simulink model "model_with_out_phases"  (R2018b)
settings: Solver=daessc  StartTime=0.0  StopTime=1  RelTol=1e-3
StopFcn:
  | % fault_type = 1005;
  | % location = 50;
  | % current = c(:,2:4);
  | % current(:,4) = fault_type;
  | % current(:,5) = location;
  | % voltage = v(:,2:4);
  | % logg = [voltage,current];
  | % data = xlsread('sdata1');
  | % data = [data;logg];
  | % xlswrite('sdata1',data);
libraries: powerlib x7, powerlib_meascontrol x2
settings Model: Creator=Edagotti Pavankumar  LastModifiedBy=Edagotti Pavankumar
settings SolverCC: ZeroCrossAlgorithm=Adaptive
settings DebuggingCC: IgnoredZcDiagnostic=none

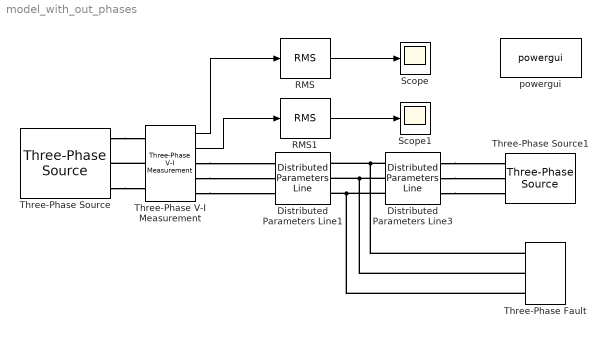
== system model_with_out_phases ==
  Distributed Parameters Line1 : powerlib/Elements/Distributed Parameters Line  Phases=3  Frequency=50  Resistance=[0.0238 0.3885]  Inductance=[0.0009509508 0.0032508989]  Capacitance=[12.74e-9 7.751e-9]  Length=50  x1=[5.84979752376728e-10 272937.603824644 272937.603824645;314.159265358979 314.159265358979 314.159265358979;1.5916152008636 0.434043679615579 -1.13675264717932]  x2=[6.54876606015739e-10 274167.064757833 274167.064757835;314.159265358979 314.159265358979 314.159265358979;1.48083589447483 0.433676655897658 -1.13711967089724]  x3=[3.33089663188176e-12 1001.56472405766 1001.56472405766;314.159265358979 314.159265358979 314.159265358979;0.373520113239949 0.324556739532956 -1.24623958726195]  x4=[1.36362276955881e-12 1001.88717060073 1001.88717060074;314.159265358979 314.159265358979 314.159265358979;2.72800603785052 0.488402443149095 -1.0823938836458]  x5=0.000250986639952707  V1=[5.85e-10 2.729e+05 2.729e+05;314.2 314.2 314.2;1.592 0.434 -1.137]  V2=[6.549e-10 2.742e+05 2.742e+05;314.2 314.2 314.2;1.481 0.4337 -1.137]  I1=[3.331e-12 1002 1002;314.2 314.2 314.2;0.3735 0.3246 -1.246]  I2=[1.364e-12 1002 1002;314.2 314.2 314.2;2.728 0.4884 -1.082]  nHarmo=1  Measurements=None
      settings: SourceProductName=Simscape Power Systems
  Distributed Parameters Line3 : powerlib/Elements/Distributed Parameters Line  Phases=3  Frequency=50  Resistance=[0.0238 0.3885]  Inductance=[0.0009509508 0.0032508989]  Capacitance=[12.74e-9 7.751e-9]  Length=150  x1=[6.54836185276508e-10 274167.064757833 274167.064757835;314.159265358979 314.159265358979 314.159265358979;1.33424699152751 0.324327959298449 -1.24646836749645]  x2=[4.51637157030593e-10 272937.917712324 272937.917712326;314.159265358979 314.159265358979 314.159265358979;1.38259637817942 0.324708516630807 -1.24608781016409]  x3=[1.33691802850131e-12 995.345525673913 995.345525673921;314.159265358979 314.159265358979 314.159265358979;2.24934769208087 0.269481792955064 -1.30131453383983]  x4=[1.38546021515408e-12 995.079620101291 995.079620101296;314.159265358979 314.159265358979 314.159265358979;0.604347333375782 0.214986476792087 -1.35580985000282]  x5=0.000752959919858122  V1=[6.548e-10 2.742e+05 2.742e+05;314.2 314.2 314.2;1.334 0.3243 -1.246]  V2=[4.516e-10 2.729e+05 2.729e+05;314.2 314.2 314.2;1.383 0.3247 -1.246]  I1=[1.337e-12 995.3 995.3;314.2 314.2 314.2;2.249 0.2695 -1.301]  I2=[1.385e-12 995.1 995.1;314.2 314.2 314.2;0.6043 0.215 -1.356]  nHarmo=1  Measurements=None
      settings: SourceProductName=Simscape Power Systems
  RMS : powerlib_meascontrol/Measurements/RMS  TrueRMS=on  Freq=50  RMSInit=0  Ts=0
  RMS1 : powerlib_meascontrol/Measurements/RMS  TrueRMS=on  Freq=50  RMSInit=0  Ts=0
  Scope : Scope
  Scope1 : Scope
  Three-Phase V-I Measurement : powerlib/Measurements/Three-Phase V-I Measurement  VoltageMeasurement=phase-to-ground  SetLabelV=off  LabelV=Vabc  Vpu=on  VpuLL=off  CurrentMeasurement=yes  SetLabelI=off  LabelI=Iabc  Ipu=on  Pbase=100e6  Vbase=220e3  OutputType=Complex  PhasorSimulation=off  PSBequivalent=0
  Three-Phase Fault : powerlib/Elements/Three-Phase Fault  InitialStates=0  FaultA=off  FaultB=on  FaultC=on  GroundFault=off  SwitchTimes=0.5  External=off  SwitchStatus=NaN  FaultResistance=20  GroundResistance=0.001  SnubberResistance=1e6  SnubberCapacitance=inf  Measurements=None
  Three-Phase Source : powerlib/Electrical Sources/Three-Phase Source  InternalConnection=Yg  VoltagePhases=off  Voltage=220e3  PhaseAngle=0  Voltage_phases=[25e3 25e3 25e3]/sqrt(3)  PhaseAngles_phases=[0 -120 +120]  Frequency=50  NonIdealSource=on  SpecifyImpedance=on  Resistance=0.8929  Inductance=16.58e-3  ShortCircuitLevel=100e6  BaseVoltage=220e3  XRratio=7  BusType=swing  Pref=10e3  Qref=0  Prefabc=[10e3, 10e3, 10e3]  Qrefabc=[0, 0, 0]  Qmin=-inf  Qmax=inf
  Three-Phase Source1 : powerlib/Electrical Sources/Three-Phase Source  InternalConnection=Yg  VoltagePhases=off  Voltage=220e3  PhaseAngle=0  Voltage_phases=[25e3 25e3 25e3]/sqrt(3)  PhaseAngles_phases=[0 -120 +120]  Frequency=50  NonIdealSource=on  SpecifyImpedance=on  Resistance=0.8929  Inductance=16.58e-3  ShortCircuitLevel=100e6  BaseVoltage=220e3  XRratio=7  BusType=PV  Pref=inf  Qref=0  Prefabc=[10e3, 10e3, 10e3]  Qrefabc=[0, 0, 0]  Qmin=-inf  Qmax=inf
  powergui : powerlib/powergui  Priority=1  SimulationMode=Continuous  SampleTime=50e-10  frequency=60  Iterations=50  frequencyindice=50  Pbase=100e6  ErrMax=1e-4  UnitsV=kV  UnitsW=MW  buscounter=0  FunctionMessages=off  echomessages=off  EnableUseOfTLC=off  CurrentSourceSwitches=off  DisableSnubberDevices=off  DisableRonSwitches=off  DisableVfSwitches=off  DisplayEquations=off  SolverType=Tustin/Backward Euler (TBE)  Interpol=off  ExternalGateDelay=off  methode=off  Ts=100  x0status=blocks  SPID=off  SwTol=0  HookPort=off  RestoreLinks=warning  ResistiveCurrentMeasurement=off  Frange=[0:2:500]  Ylog=off  Xlog=on  ShowGrid=off  save=off  variable=ZData  structure=0  ZoomFFT=off  StartTime=0.0  cycles=1  DisplayStyle=1  fundamental=60  FreqAxis=off  MaxFrequency=1000  frequencyindicesteady=1  RmsSteady=2  display=off
  wires:
  Three-Phase V-I Measurement/1 -> RMS/1
  RMS/1 -> Scope/1
  RMS1/1 -> Scope1/1
  Three-Phase V-I Measurement/2 -> RMS1/1
  connections:
  Three-Phase V-I Measurement/LConn2 -- Three-Phase Source/RConn2
  Three-Phase Source/RConn1 -- Three-Phase V-I Measurement/LConn1
  Three-Phase Source/RConn3 -- Three-Phase V-I Measurement/LConn3
  Three-Phase V-I Measurement/RConn1 -- Distributed Parameters Line1/LConn1
  Three-Phase V-I Measurement/RConn2 -- Distributed Parameters Line1/LConn2
  Three-Phase V-I Measurement/RConn3 -- Distributed Parameters Line1/LConn3
  Distributed Parameters Line3/RConn1 -- Three-Phase Source1/RConn1
  Distributed Parameters Line3/RConn2 -- Three-Phase Source1/RConn2
  Distributed Parameters Line3/RConn3 -- Three-Phase Source1/RConn3
  Distributed Parameters Line3/LConn1 -- Three-Phase Fault/LConn1 -- Distributed Parameters Line1/RConn1
  Distributed Parameters Line3/LConn2 -- Three-Phase Fault/LConn2 -- Distributed Parameters Line1/RConn2
  Distributed Parameters Line3/LConn3 -- Three-Phase Fault/LConn3 -- Distributed Parameters Line1/RConn3
